simulink model "hoffmannFollowerWPI"  (R2016b)
settings: Solver=FixedStepAuto  StartTime=0.0  StopTime=inf  FixedStep=0.025  RelTol=1e-3  EnableMultiTasking=on
model workspace (MAT data in the model file):
  SL_ROS_VariableLengthArrays_MaxSizes.CommonInfo.ArrayTruncateAction = 'EmitWarning'
  SL_ROS_VariableLengthArrays_MaxSizes.MsgTypeMap = containers.Map
  SL_ROS_VariableLengthArrays_MaxSizes.MsgTypeMap.serialization.keys = {'nav_msgs/Path'}
  SL_ROS_VariableLengthArrays_MaxSizes.MsgTypeMap.serialization.values{1}.PropertyName = 'Poses'
  SL_ROS_VariableLengthArrays_MaxSizes.MsgTypeMap.serialization.values{1}.DataType = 'geometry_msgs/PoseStamped'
  SL_ROS_VariableLengthArrays_MaxSizes.MsgTypeMap.serialization.values{1}.MaxLength = 256
  SL_ROS_VariableLengthArrays_MaxSizes.MsgTypeMap.serialization.uniformity = 0
  SL_ROS_VariableLengthArrays_MaxSizes.MsgTypeMap.serialization.keyType = 'char'
  SL_ROS_VariableLengthArrays_MaxSizes.MsgTypeMap.serialization.valueType = 'any'
undefined symbols (not defined in the file): Angular, ki, kp, kv, Linear, Pose
libraries: robotlib x12, simulink x1
settings Model: Creator=sprinkle  LastModifiedBy=nolan
settings DataIOCC: LimitDataPoints=on  ReturnWorkspaceOutputs=on
settings OptimizationCC: LifeSpan=Inf  MaxStackSize=64
settings DebuggingCC: ReadBeforeWriteMsg=DisableAll  WriteAfterWriteMsg=DisableAll  WriteAfterReadMsg=DisableAll  MultiTaskDSMMsg=none  AllowSymbolicDim=off  SFUnexpectedBacktrackingDiag=warning  SFNoUnconditionalDefaultTransitionDiag=warning  SFExecutionAtInitializationDiag=none
settings HardwareCC: ProdBitPerPointer=32  ProdBitPerSizeT=32  ProdBitPerPtrDiffT=32  ProdLargestAtomicFloat=None  ProdIntDivRoundTo=Undefined  ProdEndianess=Unspecified  ProdWordSize=32  ProdHWDeviceType=Generic->Unspecified (assume 32-bit Generic)
settings ModelReferenceCC: UpdateModelReferenceTargets=IfOutOfDate  PropagateSignalLabelsOutOfModel=off
settings SFSimCC: SFSimEcho=off
settings RTWCC: SystemTargetFile=ert.tlc  HardwareBoard=Robot Operating System (ROS)  TLCOptions=-aInlineSetEventsForThisBaseRateFcn=TLC_FALSE -aSuppressMultiTaskScheduler=TLC_FALSE -aRateBasedStepFcn=0  TemplateMakefile=ert_default_tmf  Description=Embedded Coder  GenerateReport=on  Toolchain=Catkin  BuildConfiguration=Faster Runs  LaunchReport=on  TargetLang=C++
settings CodeAppCC: ForceParamTrailComments=on  OperatorAnnotations=on  MATLABSourceComments=on
settings ERTTargetCC: ERTCustomFileBanners=off  SupportContinuousTime=on  SupportNonInlinedSFcns=on  RemoveResetFunc=off  ModelStepFunctionPrototypeControlCompliant=off
settings ConfigComp: CovMetricSettings=dw  CovHtmlReporting=on  CovSaveCumulativeToWorkspaceVar=on  CovSaveSingleToWorkspaceVar=on  CovExternalEMLEnable=off

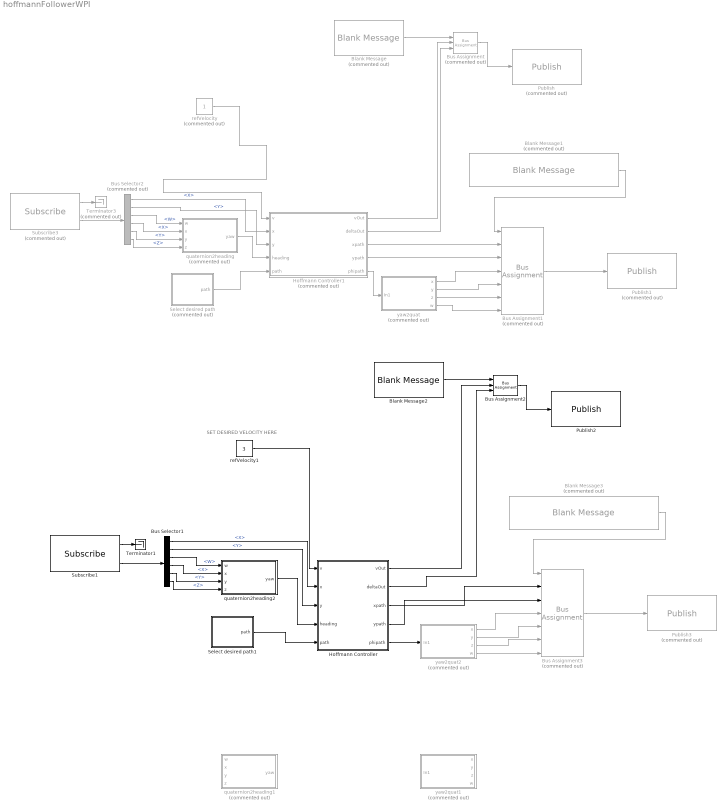
== system hoffmannFollowerWPI ==
  note: SET DESIRED VELOCITY HERE
  Blank Message : robotlib/Blank Message  Commented=on  SourceLibraryInfo=This block requires Robotics System Toolbox  messageType=geometry_msgs/Twist  SampleTime=inf
  Blank Message1 : robotlib/Blank Message  Commented=on  SourceLibraryInfo=This block requires Robotics System Toolbox  messageType=visualization_msgs/InteractiveMarkerPose  SampleTime=inf
  Blank Message2 : robotlib/Blank Message  SourceLibraryInfo=This block requires Robotics System Toolbox  messageType=geometry_msgs/Twist  SampleTime=inf
  Blank Message3 : robotlib/Blank Message  Commented=on  SourceLibraryInfo=This block requires Robotics System Toolbox  messageType=visualization_msgs/InteractiveMarkerPose  SampleTime=inf
  Bus Assignment : BusAssignment  Commented=on  AssignedSignals=Linear.X,Angular.Z
  Bus Assignment1 : BusAssignment  Commented=on  AssignedSignals=Pose.Position.X,Pose.Position.Y,Pose.Orientation.X,Pose.Orientation.Y,Pose.Orientation.Z,Pose.Orientation.W
  Bus Assignment2 : BusAssignment  AssignedSignals=Linear.X,Angular.Z
  Bus Assignment3 : BusAssignment  Commented=on  AssignedSignals=Pose.Position.X,Pose.Position.Y,Pose.Orientation.X,Pose.Orientation.Y,Pose.Orientation.Z,Pose.Orientation.W
  Bus Selector1 : BusSelector  OutputSignals=Pose.Pose.Position.X,Pose.Pose.Position.Y,Pose.Pose.Orientation.W,Pose.Pose.Orientation.X,Pose.Pose.Orientation.Y,Pose.Pose.Orientation.Z
  Bus Selector2 : BusSelector  Commented=on  OutputSignals=Pose.Pose.Position.X,Pose.Pose.Position.Y,Pose.Pose.Orientation.W,Pose.Pose.Orientation.X,Pose.Pose.Orientation.Y,Pose.Pose.Orientation.Z
  Hoffmann Controller : Subsystem
  Hoffmann Controller1 : Subsystem  Commented=on
  Publish : robotlib/Publish  Commented=on  SourceLibraryInfo=This block requires Robotics System Toolbox  topicSource=Select from ROS network  topic=/azcar_sim/cmd_vel  messageType=geometry_msgs/Twist  messageQueueLength=1
  Publish1 : robotlib/Publish  Commented=on  SourceLibraryInfo=This block requires Robotics System Toolbox  topicSource=Specify your own  topic=/azcar_sim/waypoint  messageType=visualization_msgs/InteractiveMarkerPose  messageQueueLength=1
  Publish2 : robotlib/Publish  SourceLibraryInfo=This block requires Robotics System Toolbox  topicSource=Select from ROS network  topic=/azcar_sim/cmd_vel  messageType=geometry_msgs/Twist  messageQueueLength=1
  Publish3 : robotlib/Publish  Commented=on  SourceLibraryInfo=This block requires Robotics System Toolbox  topicSource=Specify your own  topic=/azcar_sim/waypoint  messageType=visualization_msgs/InteractiveMarkerPose  messageQueueLength=1
  Select desired path : Subsystem  Commented=on
  Select desired path1 : Subsystem
  Subscribe1 : robotlib/Subscribe  SourceLibraryInfo=This block requires Robotics System Toolbox  topicSource=Select from ROS network  topic=/azcar_sim/odom  messageType=nav_msgs/Odometry  sampleTime=-1  messageQueueLength=1
  Subscribe3 : robotlib/Subscribe  Commented=on  SourceLibraryInfo=This block requires Robotics System Toolbox  topicSource=Select from ROS network  topic=/azcar_sim/odom  messageType=nav_msgs/Odometry  sampleTime=-1  messageQueueLength=1
  Terminator1 : Terminator
  Terminator3 : Terminator  Commented=on
  quaternion2heading : Subsystem  Commented=on
  quaternion2heading1 : Subsystem  Commented=on
  quaternion2heading2 : Subsystem
  refVelocity : Constant  Commented=on
  refVelocity1 : Constant  Value=3
  yaw2quat : Subsystem  Commented=on
  yaw2quat1 : Subsystem  Commented=on
  yaw2quat2 : Subsystem  Commented=on
  wires:
  Blank Message/1 -> Bus Assignment/1
  Bus Assignment/1 -> Publish/1
  Subscribe3/1 -> Terminator3/1
  Subscribe3/2 -> Bus Selector2/1
  refVelocity/1 -> Hoffmann Controller1/1(v)
  Bus Selector2/1 -> Hoffmann Controller1/2(x)  "<X>"
  Bus Selector2/2 -> Hoffmann Controller1/3(y)  "<Y>"
  Blank Message1/1 -> Bus Assignment1/1
  Bus Assignment1/1 -> Publish1/1
  yaw2quat/1(x) -> Bus Assignment1/4
  yaw2quat/2(y) -> Bus Assignment1/5
  yaw2quat/3(z) -> Bus Assignment1/6
  yaw2quat/4(w) -> Bus Assignment1/7
  Select desired path/1(path) -> Hoffmann Controller1/5(path)
  quaternion2heading/1(yaw) -> Hoffmann Controller1/4(heading)
  Bus Selector2/3 -> quaternion2heading/1(w)  "<W>"
  Bus Selector2/4 -> quaternion2heading/2(x)  "<X>"
  Bus Selector2/5 -> quaternion2heading/3(y)  "<Y>"
  Bus Selector2/6 -> quaternion2heading/4(z)  "<Z>"
  Hoffmann Controller1/5(phipath) -> yaw2quat/1(In1)
  Hoffmann Controller1/4(ypath) -> Bus Assignment1/3
  Hoffmann Controller1/3(xpath) -> Bus Assignment1/2
  Hoffmann Controller1/2(deltaOut) -> Bus Assignment/3
  Hoffmann Controller1/1(vOut) -> Bus Assignment/2
  Blank Message2/1 -> Bus Assignment2/1
  Bus Assignment2/1 -> Publish2/1
  Subscribe1/1 -> Terminator1/1
  Subscribe1/2 -> Bus Selector1/1
  refVelocity1/1 -> Hoffmann Controller/1(v)
  Bus Selector1/1 -> Hoffmann Controller/2(x)  "<X>"
  Bus Selector1/2 -> Hoffmann Controller/3(y)  "<Y>"
  Blank Message3/1 -> Bus Assignment3/1
  Bus Assignment3/1 -> Publish3/1
  yaw2quat2/1(x) -> Bus Assignment3/4
  yaw2quat2/2(y) -> Bus Assignment3/5
  yaw2quat2/3(z) -> Bus Assignment3/6
  yaw2quat2/4(w) -> Bus Assignment3/7
  Select desired path1/1(path) -> Hoffmann Controller/5(path)
  quaternion2heading2/1(yaw) -> Hoffmann Controller/4(heading)
  Bus Selector1/3 -> quaternion2heading2/1(w)  "<W>"
  Bus Selector1/4 -> quaternion2heading2/2(x)  "<X>"
  Bus Selector1/5 -> quaternion2heading2/3(y)  "<Y>"
  Bus Selector1/6 -> quaternion2heading2/4(z)  "<Z>"
  Hoffmann Controller/1(vOut) -> Bus Assignment2/2
  Hoffmann Controller/2(deltaOut) -> Bus Assignment2/3
  Hoffmann Controller/3(xpath) -> Bus Assignment3/2
  Hoffmann Controller/4(ypath) -> Bus Assignment3/3
  Hoffmann Controller/5(phipath) -> yaw2quat2/1(In1)

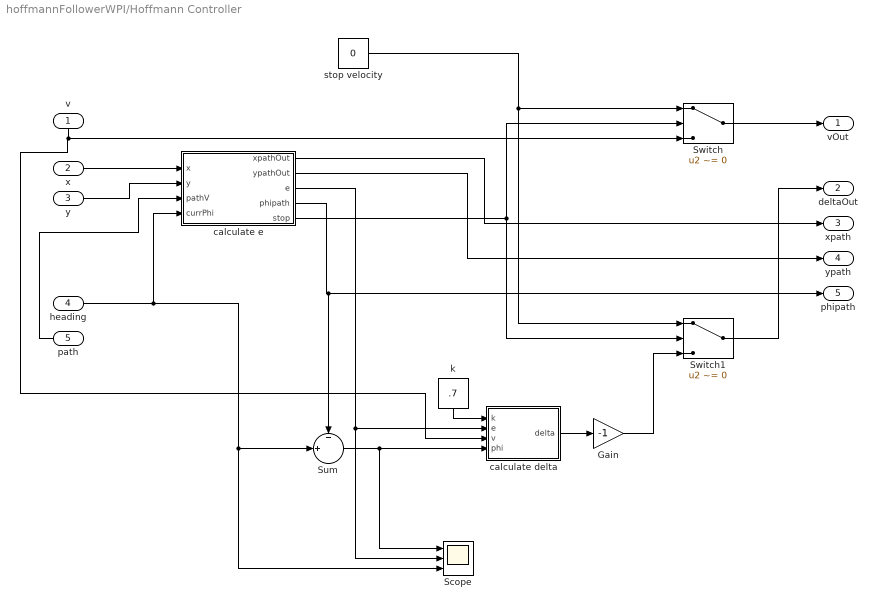
== system hoffmannFollowerWPI/Hoffmann Controller ==
  v : Inport
  x : Inport  Port=2
  y : Inport  Port=3
  heading : Inport  Port=4
  path : Inport  Port=5
  Gain : Gain  Gain=-1
  Scope : Scope  NumInputPorts=3
  Sum : Sum  Inputs=-|+||
  Switch : Switch  Criteria=u2 ~= 0  Threshold=1000  ZeroCross=off
  Switch1 : Switch  Criteria=u2 ~= 0  Threshold=1000  ZeroCross=off
  calculate delta : MATLAB Function  TreatAsAtomicUnit=on
  calculate e : MATLAB Function  TreatAsAtomicUnit=on
  k : Constant  Value=.7
  stop velocity : Constant  Value=0
  vOut : Outport
  deltaOut : Outport  Port=2
  xpath : Outport  Port=3
  ypath : Outport  Port=4
  phipath : Outport  Port=5
  wires:
  v/1 -> calculate delta/3(v), Switch/3
  path/1 -> calculate e/3(pathV)
  x/1 -> calculate e/1(x)
  y/1 -> calculate e/2(y)
  calculate e/3(e) -> calculate delta/2(e), Scope/2
  Sum/1 -> Scope/1, calculate delta/4(phi)
  k/1 -> calculate delta/1(k)
  calculate e/1(xpathOut) -> xpath/1
  calculate e/2(ypathOut) -> ypath/1
  Switch/1 -> vOut/1
  heading/1 -> Sum/2, Scope/3, calculate e/4(currPhi)
  calculate delta/1(delta) -> Gain/1
  calculate e/5(stop) -> Switch1/2, Switch/2
  calculate e/4(phipath) -> phipath/1, Sum/1
  stop velocity/1 -> Switch1/1, Switch/1
  Gain/1 -> Switch1/3
  Switch1/1 -> deltaOut/1

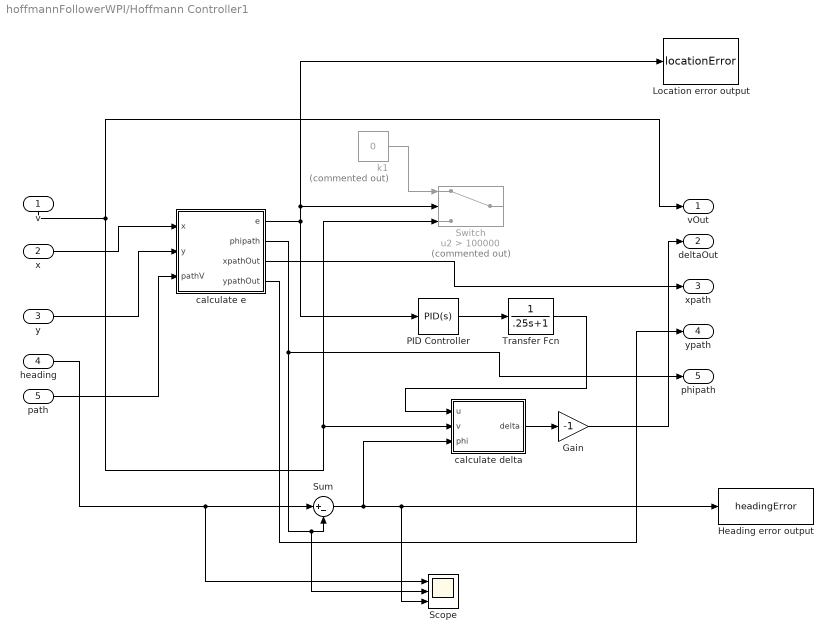
== system hoffmannFollowerWPI/Hoffmann Controller1 ==
  v : Inport
  x : Inport  Port=2
  y : Inport  Port=3
  heading : Inport  Port=4
  path : Inport  Port=5
  Gain : Gain  Gain=-1
  Heading error output : ToWorkspace  VariableName=headingError  SaveFormat=Structure With Time  SampleTime=-1
      settings: Save2DSignal=2-D array (concatenate along first dimension)
  "Location error output " : ToWorkspace  VariableName=locationError  SaveFormat=Structure With Time  SampleTime=-1
      settings: Save2DSignal=2-D array (concatenate along first dimension)
  PID Controller : simulink/Continuous/PID Controller  Controller=PID  TimeDomain=Continuous-time  SampleTime=-1  IntegratorMethod=Forward Euler  FilterMethod=Forward Euler  Form=Parallel  UseFilter=on  ControllerParametersSource=internal  P=kp  I=ki  D=kv  N=100  InitialConditionSource=internal  InitialConditionForIntegrator=0  InitialConditionForFilter=0  ExternalReset=none  LimitOutput=off  UpperSaturationLimit=inf  LowerSaturationLimit=-inf  LinearizeAsGain=on  AntiWindupMode=none  Kb=1  TrackingMode=off  Kt=1  PParamMin=[]  PParamMax=[]  IParamMin=[]  IParamMax=[]  DParamMin=[]  DParamMax=[]  NParamMin=[]  NParamMax=[]  KbParamMin=[]  KbParamMax=[]  KtParamMin=[]  KtParamMax=[]  POutMin=[]  POutMax=[]  IOutMin=[]  IOutMax=[]  DOutMin=[]  DOutMax=[]  NOutMin=[]  NOutMax=[]  KbOutMin=[]  KbOutMax=[]  KtOutMin=[]  KtOutMax=[]  IntegratorOutMin=[]  IntegratorOutMax=[]  FilterOutMin=[]  FilterOutMax=[]  SumOutMin=[]  SumOutMax=[]  SumI1OutMin=[]  SumI1OutMax=[]  SumI2OutMin=[]  SumI2OutMax=[]  SumI3OutMin=[]  SumI3OutMax=[]  SumDOutMin=[]  SumDOutMax=[]  SaturationOutMin=[]  SaturationOutMax=[]  IntegratorContinuousStateAttributes=''  IntegratorStateMustResolveToSignalObject=off  IntegratorRTWStateStorageClass=Auto  FilterContinuousStateAttributes=''  FilterStateMustResolveToSignalObject=off  FilterRTWStateStorageClass=Auto  DifferentiatorICPrevScaledInput=0  DifferentiatorOutMin=[]  DifferentiatorOutMax=[]
  Scope : Scope  NumInputPorts=3
  Sum : Sum  Inputs=|+-
  Switch : Switch  Commented=on  Criteria=u2 > Threshold  Threshold=100000
  Transfer Fcn : TransferFcn  Denominator=[.25 1]
  calculate delta : MATLAB Function  TreatAsAtomicUnit=on
  calculate e : MATLAB Function  TreatAsAtomicUnit=on
  k1 : Constant  Commented=on  Value=0
  vOut : Outport
  deltaOut : Outport  Port=2
  xpath : Outport  Port=3
  ypath : Outport  Port=4
  phipath : Outport  Port=5
  wires:
  v/1 -> Switch/3, calculate delta/2(v), vOut/1
  path/1 -> calculate e/3(pathV)
  x/1 -> calculate e/1(x)
  y/1 -> calculate e/2(y)
  calculate e/2(phipath) -> phipath/1, Scope/2, Sum/2
  calculate e/1(e) -> "Location error output "/1, Switch/2, PID Controller/1
  Sum/1 -> calculate delta/3(phi), Scope/3, Heading error output/1
  calculate e/3(xpathOut) -> xpath/1
  calculate e/4(ypathOut) -> ypath/1
  k1/1 -> Switch/1
  heading/1 -> Scope/1, Sum/1
  calculate delta/1(delta) -> Gain/1
  Gain/1 -> deltaOut/1
  PID Controller/1 -> Transfer Fcn/1
  Transfer Fcn/1 -> calculate delta/1(u)

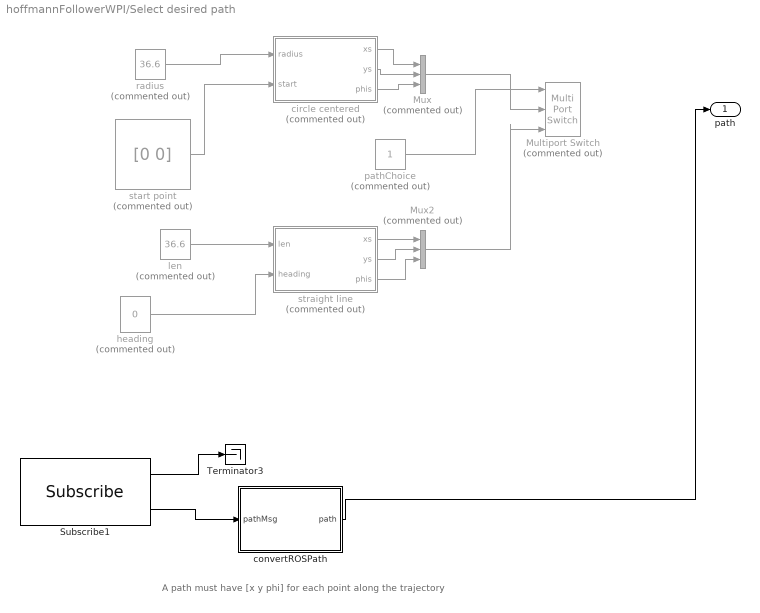
== system hoffmannFollowerWPI/Select desired path ==
  note: A path must have [x y phi] for each point along the trajectory
  Multiport Switch : MultiPortSwitch  Commented=on  Inputs=2
  Mux : Mux  Commented=on  Inputs=3
  Mux2 : Mux  Commented=on  Inputs=3
  Subscribe1 : robotlib/Subscribe  SourceLibraryInfo=This block requires Robotics System Toolbox  topicSource=Select from ROS network  topic=/path  messageType=nav_msgs/Path  sampleTime=-1  messageQueueLength=1
  Terminator3 : Terminator
  circle centered : MATLAB Function  Commented=on  TreatAsAtomicUnit=on
  convertROSPath : MATLAB Function  TreatAsAtomicUnit=on
  heading : Constant  Commented=on  Value=0
  len : Constant  Commented=on  Value=36.6
  "pathChoice " : Constant  Commented=on
  radius : Constant  Commented=on  Value=36.6
  start point : Constant  Commented=on  Value=[0 0]
  straight line : MATLAB Function  Commented=on  TreatAsAtomicUnit=on
  path : Outport
  wires:
  radius/1 -> circle centered/1(radius)
  start point/1 -> circle centered/2(start)
  "pathChoice "/1 -> Multiport Switch/1
  circle centered/2(ys) -> Mux/2
  circle centered/1(xs) -> Mux/1
  len/1 -> straight line/1(len)
  heading/1 -> straight line/2(heading)
  straight line/1(xs) -> Mux2/1
  straight line/2(ys) -> Mux2/2
  Mux2/1 -> Multiport Switch/3
  Mux/1 -> Multiport Switch/2
  straight line/3(phis) -> Mux2/3
  circle centered/3(phis) -> Mux/3
  Subscribe1/2 -> convertROSPath/1(pathMsg)
  convertROSPath/1(path) -> path/1
  Subscribe1/1 -> Terminator3/1

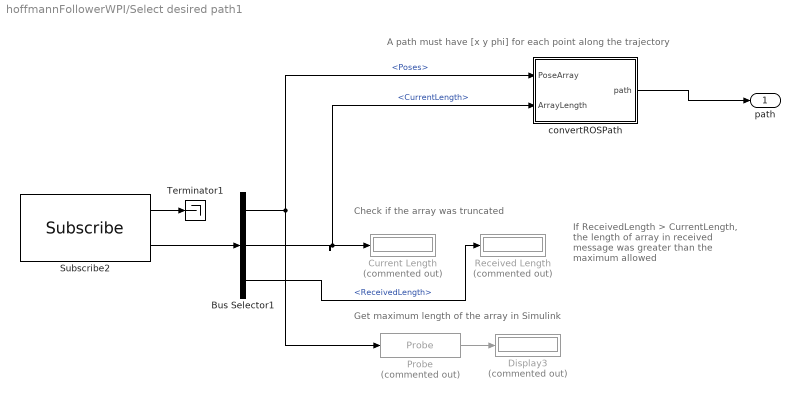
== system hoffmannFollowerWPI/Select desired path1 ==
  note: A path must have [x y phi] for each point along the trajectory
  note: If ReceivedLength > CurrentLength, the length of array in received message was greater than the maximum allowed
  note: Check if the array was truncated
  note: Get maximum length of the array in Simulink
  Bus Selector1 : BusSelector  OutputSignals=Poses,Poses_SL_Info.CurrentLength,Poses_SL_Info.ReceivedLength
  Current Length : Display  Commented=on
  Display3 : Display  Commented=on
  Probe : Probe  Commented=on  ProbeWidth=off  ProbeSampleTime=off  ProbeComplexSignal=off  ProbeSignalDimensions=on
  Received Length : Display  Commented=on
  Subscribe2 : robotlib/Subscribe  SourceLibraryInfo=This block requires Robotics System Toolbox  topicSource=Specify your own  topic=/path  messageType=nav_msgs/Path  sampleTime=0.025  messageQueueLength=1
  Terminator1 : Terminator
  convertROSPath : MATLAB Function  TreatAsAtomicUnit=on
  path : Outport
  wires:
  convertROSPath/1(path) -> path/1
  Subscribe2/2 -> Bus Selector1/1
  Subscribe2/1 -> Terminator1/1
  Bus Selector1/1 -> convertROSPath/1(PoseArray), Probe/1  "<Poses>"
  Bus Selector1/2 -> convertROSPath/2(ArrayLength), Current Length/1  "<CurrentLength>"
  Probe/1 -> Display3/1
  Bus Selector1/3 -> Received Length/1  "<ReceivedLength>"

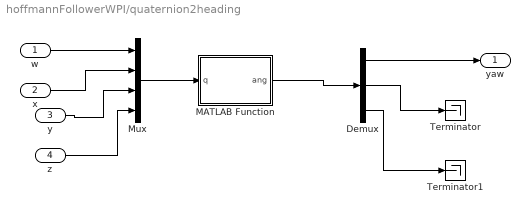
== system hoffmannFollowerWPI/quaternion2heading ==
  w : Inport
  x : Inport  Port=2
  y : Inport  Port=3
  z : Inport  Port=4
  Demux : Demux  Outputs=3
  MATLAB Function : MATLAB Function  TreatAsAtomicUnit=on
  Mux : Mux
  Terminator : Terminator
  Terminator1 : Terminator
  yaw : Outport
  wires:
  MATLAB Function/1(ang) -> Demux/1
  Demux/2 -> Terminator/1
  Demux/3 -> Terminator1/1
  Demux/1 -> yaw/1
  w/1 -> Mux/1
  x/1 -> Mux/2
  y/1 -> Mux/3
  z/1 -> Mux/4
  Mux/1 -> MATLAB Function/1(q)

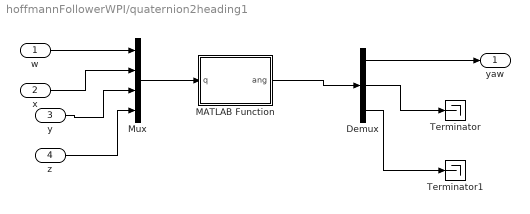
== system hoffmannFollowerWPI/quaternion2heading1 ==
  w : Inport
  x : Inport  Port=2
  y : Inport  Port=3
  z : Inport  Port=4
  Demux : Demux  Outputs=3
  MATLAB Function : MATLAB Function  TreatAsAtomicUnit=on
  Mux : Mux
  Terminator : Terminator
  Terminator1 : Terminator
  yaw : Outport
  wires:
  MATLAB Function/1(ang) -> Demux/1
  Demux/2 -> Terminator/1
  Demux/3 -> Terminator1/1
  Demux/1 -> yaw/1
  w/1 -> Mux/1
  x/1 -> Mux/2
  y/1 -> Mux/3
  z/1 -> Mux/4
  Mux/1 -> MATLAB Function/1(q)

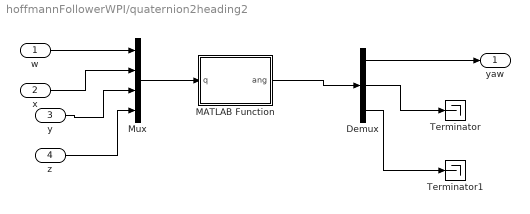
== system hoffmannFollowerWPI/quaternion2heading2 ==
  w : Inport
  x : Inport  Port=2
  y : Inport  Port=3
  z : Inport  Port=4
  Demux : Demux  Outputs=3
  MATLAB Function : MATLAB Function  TreatAsAtomicUnit=on
  Mux : Mux
  Terminator : Terminator
  Terminator1 : Terminator
  yaw : Outport
  wires:
  MATLAB Function/1(ang) -> Demux/1
  Demux/2 -> Terminator/1
  Demux/3 -> Terminator1/1
  Demux/1 -> yaw/1
  w/1 -> Mux/1
  x/1 -> Mux/2
  y/1 -> Mux/3
  z/1 -> Mux/4
  Mux/1 -> MATLAB Function/1(q)

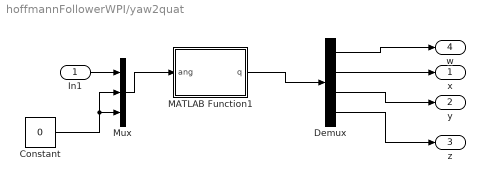
== system hoffmannFollowerWPI/yaw2quat ==
  In1 : Inport
  Constant : Constant  Value=0
  Demux : Demux
  MATLAB Function1 : MATLAB Function  TreatAsAtomicUnit=on
  Mux : Mux  Inputs=3
  x : Outport
  y : Outport  Port=2
  z : Outport  Port=3
  w : Outport  Port=4
  wires:
  Demux/1 -> w/1
  Demux/2 -> x/1
  Demux/3 -> y/1
  Demux/4 -> z/1
  In1/1 -> Mux/1
  Mux/1 -> MATLAB Function1/1(ang)
  Constant/1 -> Mux/3, Mux/2
  MATLAB Function1/1(q) -> Demux/1

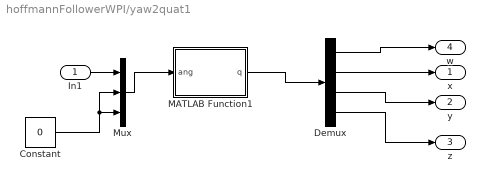
== system hoffmannFollowerWPI/yaw2quat1 ==
  In1 : Inport
  Constant : Constant  Value=0
  Demux : Demux
  MATLAB Function1 : MATLAB Function  TreatAsAtomicUnit=on
  Mux : Mux  Inputs=3
  x : Outport
  y : Outport  Port=2
  z : Outport  Port=3
  w : Outport  Port=4
  wires:
  Demux/1 -> w/1
  Demux/2 -> x/1
  Demux/3 -> y/1
  Demux/4 -> z/1
  In1/1 -> Mux/1
  Mux/1 -> MATLAB Function1/1(ang)
  Constant/1 -> Mux/3, Mux/2
  MATLAB Function1/1(q) -> Demux/1

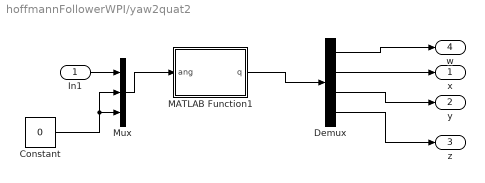
== system hoffmannFollowerWPI/yaw2quat2 ==
  In1 : Inport
  Constant : Constant  Value=0
  Demux : Demux
  MATLAB Function1 : MATLAB Function  TreatAsAtomicUnit=on
  Mux : Mux  Inputs=3
  x : Outport
  y : Outport  Port=2
  z : Outport  Port=3
  w : Outport  Port=4
  wires:
  Demux/1 -> w/1
  Demux/2 -> x/1
  Demux/3 -> y/1
  Demux/4 -> z/1
  In1/1 -> Mux/1
  Mux/1 -> MATLAB Function1/1(ang)
  Constant/1 -> Mux/3, Mux/2
  MATLAB Function1/1(q) -> Demux/1

== matlab function hoffmannFollowerWPI/Hoffmann Controller/calculate e ==
  data: xpathOut output; ypathOut output; e output; x input; y input; pathV input size=[256 3]; phipath output; stop output; currPhi input
function [xpathOut,ypathOut,e,phipath,stop] = fcn(x,y,pathV,currPhi)
%#codegen
if isempty(pathV)
    % if no path yet retain current position
    e = 0;
    phipath = currPhi;
    xpathOut = x;
    ypathOut = y;
    stop = 1;
    return
end
path=reshape(pathV,[],3);
x1 = path(1,1);
y1 = path(1,2);
phi1=path(1,3);
etmp = inf;
e = inf;
index=1;
% find the nearest x,y
for i=1:length(path)
   etmp = sqrt((x-path(i,1))^2+(y-path(i,2))^2);
   if( etmp < e )
       e = etmp;
       index=i;
   end
end

if index ==length(path)
    stop = 1;
else
    stop = 0;
end

xpathOut=path(index,1);
ypathOut=path(index,2);
phipath=path(index,3);

ex1 = (path(index,1)-x);
ey1 = (path(index,2)-y);
ex2 = cos(phipath);
ey2 = sin(phipath);
sinnnn = ex1*ey2-ey1*ex2;
e = sign(sinnnn)*e;

== matlab function hoffmannFollowerWPI/quaternion2heading/MATLAB Function ==
  data: q input; ang output
function ang = yawFromQuaternions(q)
% YAWFROMQUATERNIONS y = YAWFROMQUATERNIONS(qVect) calculates Yaw about z
% axis given a quaternion
% INPUT q - [w x y z] = [rotation, vectX, vectY, vectZ] [angle,1x3 vector]
% OUTPUT ang - radians
% see https://en.wikipedia.org/wiki/Conversion_between_quaternions_and_Euler_angles
W = q(1);
X = q(2);
Y = q(3);
Z = q(4);

ysqr = Y^2;
t0 = -2 * (ysqr + Z * Z) + 1;
t1 = +2 * (X * Y - W * Z);
t2 = -2 * (X * Z + W * Y);
t3 = +2 * (Y * Z - W * X);
t4 = -2 * (X * X + ysqr) + 1;
if t2 > 1
    t2 =1;
elseif t2 <-1
    t2 = -1;
end
pitch = asin(t2);
roll = atan2(t3, t4);
yaw = atan2(t1, t0);

ang = [yaw, pitch, roll];
end

== matlab function hoffmannFollowerWPI/Hoffmann Controller/calculate delta ==
  data: delta output; k input; e input; v input; phi input
function delta = fcn(k,e,v,phi)
%#codegen
if( abs(v) < eps )
    v = eps;
end

% if phi is greater than pi (or less than -pi), then 
% we normalize to between [-pi,pi]
if( phi < -pi )
    phi = phi+2*pi;
elseif( phi > pi )
    phi = phi-2*pi;
end

delta = phi + atan2(k*e,v);

== matlab function hoffmannFollowerWPI/Select desired path/circle centered ==
  data: xs output; radius input; start input; ys output; phis output
function [xs,ys,phis] = fcn(radius,start)
%#codegen
angles=linspace(-pi,pi,301);
r = radius*exp(angles*1j);
xs = real(r)-radius+start(1);
ys = imag(r)+start(2);
phis=(pi/2)+angles;

% % To visualize the angles, run this code:
% radius=3.6; start=[0 0];
% angles=linspace(-pi,pi,300);
% r = radius*exp(angles*1j);
% xs = real(r)-radius+start(1);
% ys = imag(r)+start(2);
% % since the direction of travel is in the 'x' direction, the 
% % heading (phi) matchines the angle of the circle
% phis=(pi/2)+angles;
% xends=cos(phis);yends=sin(phis);
% figure;plot(xs,ys);hold on; quiver(xs,ys,xends,yends);axis equal;hold off

== matlab function hoffmannFollowerWPI/Select desired path/straight line ==
  data: xs output; len input; heading input; ys output; phis output
function [xs,ys,phis] = fcn(len,heading)
%#codegen
r = linspace(0,len,301);
xs = r*cos(heading);
ys = r*sin(heading);
phis = heading*ones(1,length(r));

== matlab function hoffmannFollowerWPI/Select desired path/convertROSPath ==
  data: path output; pathMsg input
function path  = fcn(pathMsg)
%#codegen
PoseArray = pathMsg.Poses;
numPt = length(PoseArray);
xs = zeros(numPt,1);
ys = zeros(numPt,1);
phis = zeros(numPt,1);
for i = 1:numPt
    xs(i) = PoseArray(i).Pose.Position.X;
    ys(i) = PoseArray(i).Pose.Position.Y;
    qVect = PoseArray(i).Pose.Orientation;
    phis(i) = yawFromQuaternions(qVect);
end
path = [xs, ys, phis];
end

function yaw = yawFromQuaternions(q)
% YAWFROMQUATERNIONS y = YAWFROMQUATERNIONS(qVect) calculates Yaw about z
% axis given a quaternion
% INPUT q - [w x y z] = [rotation, vectX, vectY, vectZ] [angle,1x3 vector]
% OUTPUT y - yaw radians
% see https://en.wikipedia.org/wiki/Conversion_between_quaternions_and_Euler_angles
% a = q.X;
% b = q.Y;
% c = q.Z;
% d = q.W;
% N = 2*(a*d+b*c);
% D = a^2 + b^2 - c^2 -d^2;
% y = atan2(N,D);

ysqr = q.Y^2;
t0 = -2 * (ysqr + q.Z * q.Z) + 1;
t1 = +2 * (q.X * q.Y - q.W * q.Z);
t2 = -2 * (q.X * q.Z + q.W * q.Y);
t3 = +2 * (q.Y * q.Z - q.W * q.X);
t4 = -2 * (q.X * q.X + ysqr) + 1;
if t2 > 1
    t2 =1;
elseif t2 <-1
    t2 = -1;
end
pitch = asin(t2);
roll = atan2(t3, t4);
yaw = atan2(t1, t0);
end

== matlab function hoffmannFollowerWPI/yaw2quat/MATLAB Function1 ==
  data: ang input; q output
function q = yaw2quat(ang)
% YAWFROMQUATERNIONS y = YAWFROMQUATERNIONS(qVect) calculates Yaw about z
% axis given a quaternion
% INPUT ang = [y 0 0] [angle,1x3 vector]
% OUTPUT y - yaw radians
% see http://www.chrobotics.com/library/understanding-quaternions
yaw = ang(1);
roll = ang(2);
pitch = ang(3);

t0 = cos(yaw * 0.5);
t1 = sin(yaw * 0.5);
t2 = cos(roll * 0.5);
t3 = sin(roll * 0.5);
t4 = cos(pitch * 0.5);
t5 = sin(pitch * 0.5);
q = zeros(4,1);
q(4) = t0 * t2 * t4 + t1 * t3 * t5;
q(1) = t0 * t3 * t4 - t1 * t2 * t5;
q(2) = t0 * t2 * t5 + t1 * t3 * t4;
q(3) = t1 * t2 * t4 - t0 * t3 * t5;
end

== matlab function hoffmannFollowerWPI/Hoffmann Controller1/calculate delta ==
  data: delta output; u input; v input; phi input
function delta = fcn(u,v,phi)
%#codegen
if( abs(v) < eps )
    v = eps;
end

% if phi is greater than pi (or less than -pi), then 
% we normalize to between [-pi,pi]
if( phi < -pi )
    phi = phi+2*pi;
elseif( phi > pi )
    phi = phi-2*pi;
end

delta = phi + atan2(u,v);

== matlab function hoffmannFollowerWPI/Hoffmann Controller1/calculate e ==
  data: e output; x input; y input; pathV input; phipath output; xpathOut output; ypathOut output
function [e,phipath,xpathOut,ypathOut] = fcn(x,y,pathV)
%#codegen
path=reshape(pathV,[],3);
x1 = path(1,1);
y1 = path(1,2);
phi1=path(1,3);
etmp = inf;
e = inf;
index=1;
% find the nearest x,y
for i=1:length(path)
   etmp = sqrt((x-path(i,1))^2+(y-path(i,2))^2);
   if( etmp < e )
       e = etmp;
       index=i;
   end
end

xpathOut=path(index,1);
ypathOut=path(index,2);
phipath=path(index,3);

ex1 = (path(index,1)-x);
ey1 = (path(index,2)-y);
ex2 = cos(phipath);
ey2 = sin(phipath);
sinnnn = ex1*ey2-ey1*ex2;
e = sign(sinnnn)*e;

== matlab function hoffmannFollowerWPI/quaternion2heading2/MATLAB Function ==
  data: q input; ang output
function ang = yawFromQuaternions(q)
% YAWFROMQUATERNIONS y = YAWFROMQUATERNIONS(qVect) calculates Yaw about z
% axis given a quaternion
% INPUT q - [w x y z] = [rotation, vectX, vectY, vectZ] [angle,1x3 vector]
% OUTPUT ang - radians
% see https://en.wikipedia.org/wiki/Conversion_between_quaternions_and_Euler_angles
% NOTE: The above wikipedia page history shows a major edit to these
% equations between: Revision as of 09:54, 14 November 2016 and 
% revision as of 19:12, 15 December 2016

W = q(1);
X = q(2);
Y = q(3);
Z = q(4);
% roll about x axis
ysqr = Y^2;
t0 = 2 * (W * X + Y * Z);
t1 = 1 - 2 * (X * X + ysqr);
roll = atan2(t0, t1);
% pitch about Y axis
t2 = 2 * (W * Y - Z * X);
if t2 > 1
    t2 =1;
elseif t2 <-1
    t2 = -1;
end
pitch = asin(t2);
%yaw about z axis
t3 = 2 * (W * Z - X * Y);
t4 = 1 -2 * (ysqr + Z * Z);


yaw = atan2(t3, t4);

ang = [yaw, pitch, roll];
end

== matlab function hoffmannFollowerWPI/yaw2quat2/MATLAB Function1 ==
  data: ang input; q output
function q = yaw2quat(ang)
% YAWFROMQUATERNIONS y = YAWFROMQUATERNIONS(qVect) calculates Yaw about z
% axis given a quaternion
% INPUT ang = [y 0 0] [angle,1x3 vector]
% OUTPUT y - yaw radians
% see http://www.chrobotics.com/library/understanding-quaternions
yaw = ang(1);
roll = ang(2);
pitch = ang(3);

t0 = cos(yaw * 0.5);
t1 = sin(yaw * 0.5);
t2 = cos(roll * 0.5);
t3 = sin(roll * 0.5);
t4 = cos(pitch * 0.5);
t5 = sin(pitch * 0.5);
q = zeros(4,1);
q(4) = t0 * t2 * t4 + t1 * t3 * t5;
q(1) = t0 * t3 * t4 - t1 * t2 * t5;
q(2) = t0 * t2 * t5 + t1 * t3 * t4;
q(3) = t1 * t2 * t4 - t0 * t3 * t5;
end

== matlab function hoffmannFollowerWPI/Select desired path1/convertROSPath ==
  data: path output size=[256 3]; PoseArray input; ArrayLength input
function path  = fcn(PoseArray,ArrayLength)
%#codegen
if ArrayLength > 0 && ArrayLength <256
    xs = zeros(ArrayLength,1);
    ys = zeros(ArrayLength,1);
    phis = zeros(ArrayLength,1);
    for i = 1:ArrayLength
        xs(i) = PoseArray(i).Pose.Position.X;
        ys(i) = PoseArray(i).Pose.Position.Y;
        qVect = PoseArray(i).Pose.Orientation;
        phis(i) = yawFromQuaternions(qVect);
    end
    path = [xs, ys, phis];
else
    path = [];
end
end

    function yaw = yawFromQuaternions(q)
        % YAWFROMQUATERNIONS y = YAWFROMQUATERNIONS(qVect) calculates Yaw about z
        % axis given a quaternion
        % INPUT q - [w x y z] = [rotation, vectX, vectY, vectZ] [angle,1x3 vector]
        % OUTPUT y - yaw radians
        % see https://en.wikipedia.org/wiki/Conversion_between_quaternions_and_Euler_angles
        % a = q.X;
        % b = q.Y;
        % c = q.Z;
        % d = q.W;
        % N = 2*(a*d+b*c);
        % D = a^2 + b^2 - c^2 -d^2;
        % y = atan2(N,D);
        
        ysqr = q.Y^2;
        t0 = -2 * (ysqr + q.Z * q.Z) + 1;
        t1 = +2 * (q.X * q.Y - q.W * q.Z);
        t2 = -2 * (q.X * q.Z + q.W * q.Y);
        t3 = +2 * (q.Y * q.Z - q.W * q.X);
        t4 = -2 * (q.X * q.X + ysqr) + 1;
        if t2 > 1
            t2 =1;
        elseif t2 <-1
            t2 = -1;
        end
        pitch = asin(t2);
        roll = atan2(t3, t4);
        yaw = atan2(t1, t0);
    end

== matlab function hoffmannFollowerWPI/quaternion2heading1/MATLAB Function ==
  data: q input; ang output
function ang = yawFromQuaternions(q)
% YAWFROMQUATERNIONS y = YAWFROMQUATERNIONS(qVect) calculates Yaw about z
% axis given a quaternion
% INPUT q - [w x y z] = [rotation, vectX, vectY, vectZ] [angle,1x3 vector]
% OUTPUT ang - radians
% see https://en.wikipedia.org/wiki/Conversion_between_quaternions_and_Euler_angles
W = q(1);
X = q(2);
Y = q(3);
Z = q(4);

ysqr = Y^2;
t0 = -2 * (ysqr + Z * Z) + 1;
t1 = +2 * (X * Y - W * Z);
t2 = -2 * (X * Z + W * Y);
t3 = +2 * (Y * Z - W * X);
t4 = -2 * (X * X + ysqr) + 1;
if t2 > 1
    t2 =1;
elseif t2 <-1
    t2 = -1;
end
pitch = asin(t2);
roll = atan2(t3, t4);
yaw = atan2(t1, t0);

ang = [yaw, pitch, roll];
end

== matlab function hoffmannFollowerWPI/yaw2quat1/MATLAB Function1 ==
  data: ang input; q output
function q = yaw2quat(ang)
% YAWFROMQUATERNIONS y = YAWFROMQUATERNIONS(qVect) calculates Yaw about z
% axis given a quaternion
% INPUT ang = [y 0 0] [angle,1x3 vector]
% OUTPUT y - yaw radians
% see http://www.chrobotics.com/library/understanding-quaternions
yaw = ang(1);
roll = ang(2);
pitch = ang(3);

t0 = cos(yaw * 0.5);
t1 = sin(yaw * 0.5);
t2 = cos(roll * 0.5);
t3 = sin(roll * 0.5);
t4 = cos(pitch * 0.5);
t5 = sin(pitch * 0.5);
q = zeros(4,1);
q(4) = t0 * t2 * t4 + t1 * t3 * t5;
q(1) = t0 * t3 * t4 - t1 * t2 * t5;
q(2) = t0 * t2 * t5 + t1 * t3 * t4;
q(3) = t1 * t2 * t4 - t0 * t3 * t5;
end
